simulink model "CruiseControl_Perfect_TopItOffHarness"  (R2020a)
settings: configuration reference "ModelReferencingVisual" (kept outside this file)
settings Model: DataDictionary=CruiseControl_Req_dd.sldd  Creator=yleong  LastModifiedBy=promero
settings ConfigSetRef: SourceName=ModelReferencingVisual

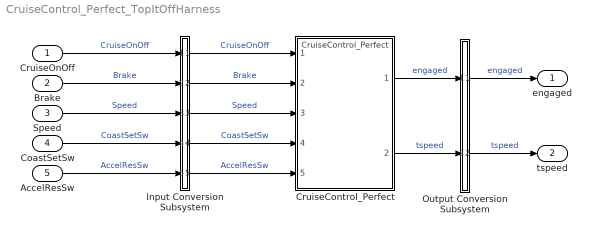
== system CruiseControl_Perfect_TopItOffHarness ==
  CruiseOnOff : Inport  OutDataTypeStr=boolean  PortDimensions=[1]  SampleTime=0.1
  Brake : Inport  Port=2  OutDataTypeStr=boolean  PortDimensions=[1]  SampleTime=0.1
  Speed : Inport  Port=3  OutDataTypeStr=uint8  PortDimensions=[1]  SampleTime=0.1
  CoastSetSw : Inport  Port=4  OutDataTypeStr=boolean  PortDimensions=[1]  SampleTime=0.1
  AccelResSw : Inport  Port=5  OutDataTypeStr=boolean  PortDimensions=[1]  SampleTime=0.1
  CruiseControl_Perfect : ModelReference  ModelNameDialog=CruiseControl_Perfect  SimulationMode=Normal  ModelReferenceVersion=1.471
  Input Conversion Subsystem : Subsystem  Tag=__SLT_ICS__  Description=|
      | Signal spec.
      | and routing
      settings: AttributesFormatString=%<Description>
  Output Conversion Subsystem : Subsystem  Tag=__SLT_OCS__  Description=|
      | Signal spec.
      | and routing
      settings: AttributesFormatString=%<Description>
  engaged : Outport
  tspeed : Outport  Port=2
  wires:
  CruiseOnOff/1 -> Input Conversion Subsystem/1(Inport_1)  "CruiseOnOff"
  Brake/1 -> Input Conversion Subsystem/2(Inport_2)  "Brake"
  Speed/1 -> Input Conversion Subsystem/3(Inport_3)  "Speed"
  CoastSetSw/1 -> Input Conversion Subsystem/4(Inport_4)  "CoastSetSw"
  AccelResSw/1 -> Input Conversion Subsystem/5(Inport_5)  "AccelResSw"
  Output Conversion Subsystem/1(Outport_1) -> engaged/1  "engaged"
  Output Conversion Subsystem/2(Outport_2) -> tspeed/1  "tspeed"
  Input Conversion Subsystem/1(Outport_1) -> CruiseControl_Perfect/1  "CruiseOnOff"
  Input Conversion Subsystem/2(Outport_2) -> CruiseControl_Perfect/2  "Brake"
  Input Conversion Subsystem/3(Outport_3) -> CruiseControl_Perfect/3  "Speed"
  Input Conversion Subsystem/4(Outport_4) -> CruiseControl_Perfect/4  "CoastSetSw"
  Input Conversion Subsystem/5(Outport_5) -> CruiseControl_Perfect/5  "AccelResSw"
  CruiseControl_Perfect/1 -> Output Conversion Subsystem/1(Inport_1)  "engaged"
  CruiseControl_Perfect/2 -> Output Conversion Subsystem/2(Inport_2)  "tspeed"

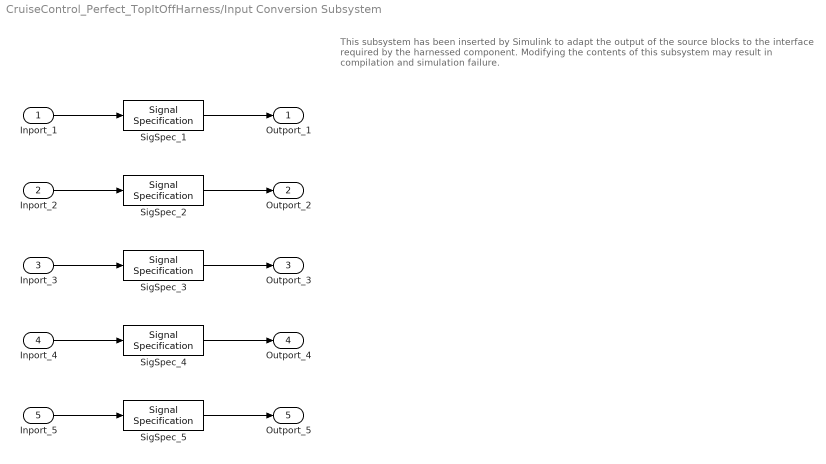
== system CruiseControl_Perfect_TopItOffHarness/Input Conversion Subsystem ==
  note: This subsystem has been inserted by Simulink to adapt the output of the source blocks to the interface required by the harnessed component.
      |  Modifying the contents of this subsystem may result in compilation and simulation failure.
  Inport_1 : Inport
  Inport_2 : Inport  Port=2
  Inport_3 : Inport  Port=3
  Inport_4 : Inport  Port=4
  Inport_5 : Inport  Port=5
  SigSpec_{1..2,4..5} (4 alike) : SignalSpecification  OutDataTypeStr=boolean  Dimensions=[1]  SampleTime=0.1
  SigSpec_3 : SignalSpecification  OutDataTypeStr=uint8  Dimensions=[1]  SampleTime=0.1
  Outport_1 : Outport
  Outport_2 : Outport  Port=2
  Outport_3 : Outport  Port=3
  Outport_4 : Outport  Port=4
  Outport_5 : Outport  Port=5
  wires:
  SigSpec_1/1 -> Outport_1/1
  Inport_1/1 -> SigSpec_1/1
  SigSpec_2/1 -> Outport_2/1
  Inport_2/1 -> SigSpec_2/1
  SigSpec_3/1 -> Outport_3/1
  Inport_3/1 -> SigSpec_3/1
  SigSpec_4/1 -> Outport_4/1
  Inport_4/1 -> SigSpec_4/1
  SigSpec_5/1 -> Outport_5/1
  Inport_5/1 -> SigSpec_5/1

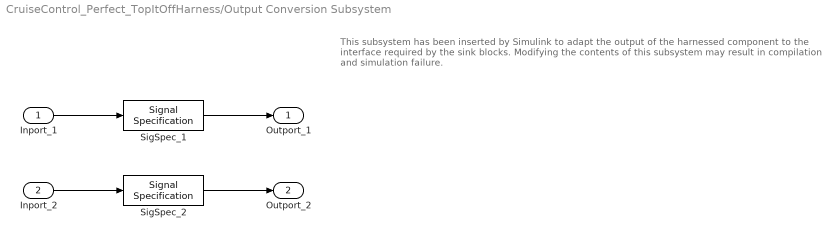
== system CruiseControl_Perfect_TopItOffHarness/Output Conversion Subsystem ==
  note: This subsystem has been inserted by Simulink to adapt the output of the harnessed component to the interface required by the sink blocks.
      |  Modifying the contents of this subsystem may result in compilation and simulation failure.
  Inport_1 : Inport
  Inport_2 : Inport  Port=2
  SigSpec_1 : SignalSpecification  OutDataTypeStr=boolean  Dimensions=[1]  SampleTime=0.1
  SigSpec_2 : SignalSpecification  OutDataTypeStr=uint8  Dimensions=[1]  SampleTime=0.1
  Outport_1 : Outport
  Outport_2 : Outport  Port=2
  wires:
  Inport_1/1 -> SigSpec_1/1
  SigSpec_1/1 -> Outport_1/1
  Inport_2/1 -> SigSpec_2/1
  SigSpec_2/1 -> Outport_2/1
